simulink model "case7"  (R2024b)
settings: Solver=FixedStepAuto  StartTime=0  StopTime=1  FixedStep=1e-7  RelTol=1e-3
values from neighbouring files (symbols this model uses):
  SG_D_1_D = 0.01056    [IEEE9_case_parameters.m]    (also in case1_parameters.m; case2_parameters.m; case3_parameters.m; case4_parameters.m)
  SG_D_1_EnableSaturation = 0    [IEEE9_case_parameters.m]    (also in case1_parameters.m; case2_parameters.m; case3_parameters.m; case4_parameters.m)
  SG_D_1_f0 = 60    [IEEE9_case_parameters.m]    (also in case1_parameters.m; case2_parameters.m; case3_parameters.m; case4_parameters.m)
  SG_D_1_H = 7.5    [IEEE9_case_parameters.m]    (also in case1_parameters.m; case2_parameters.m; case3_parameters.m; case4_parameters.m)
  SG_D_1_K_A = 20    [IEEE9_case_parameters.m]    (also in case1_parameters.m; case2_parameters.m; case3_parameters.m; case4_parameters.m)
  SG_D_1_K_E = 1.000000e+1    (= 10)    [IEEE9_case_parameters.m]    (also in case1_parameters.m; case2_parameters.m; case3_parameters.m; case4_parameters.m)
  SG_D_1_K_F = 2.363    [IEEE9_case_parameters.m]    (also in case1_parameters.m; case2_parameters.m; case3_parameters.m; case4_parameters.m)
  SG_D_1_K_s = 0.5    [IEEE9_case_parameters.m]    (also in case1_parameters.m = 5; case2_parameters.m = 5; case3_parameters.m = 5; case4_parameters.m = 5)
  SG_D_1_R_a = 0.001088    [IEEE9_case_parameters.m]    (also in case1_parameters.m; case2_parameters.m; case3_parameters.m; case4_parameters.m)
  SG_D_1_S_A = 1    [IEEE9_case_parameters.m]    (also in case1_parameters.m; case2_parameters.m; case3_parameters.m; case4_parameters.m)
  SG_D_1_S_B = 0.103    [IEEE9_case_parameters.m]    (also in case1_parameters.m; case2_parameters.m; case3_parameters.m; case4_parameters.m)
  SG_D_1_S_N = 10.659857    [IEEE9_case_parameters.m]    (also in case1_parameters.m; case2_parameters.m; case3_parameters.m; case4_parameters.m)
  SG_D_1_SpeedPara = 200    [IEEE9_case_parameters.m]    (also in case1_parameters.m; case2_parameters.m; case3_parameters.m; case4_parameters.m)
  SG_D_1_T_0 = 0.720173    [IEEE9_case_parameters.m]    (also in case1_parameters.m = 0.755522; case2_parameters.m = 0.808931; case3_parameters.m = 0.869402; case4_parameters.m = 0.729316)
  SG_D_1_T_1 = 0.3    [IEEE9_case_parameters.m]    (also in case1_parameters.m; case2_parameters.m; case3_parameters.m; case4_parameters.m)
  SG_D_1_T_2 = 0.05    [IEEE9_case_parameters.m]    (also in case1_parameters.m; case2_parameters.m; case3_parameters.m; case4_parameters.m)
  SG_D_1_T_3 = 0.02    [IEEE9_case_parameters.m]    (also in case1_parameters.m; case2_parameters.m; case3_parameters.m; case4_parameters.m)
  SG_D_1_T_4 = 0.005    [IEEE9_case_parameters.m]    (also in case1_parameters.m; case2_parameters.m; case3_parameters.m; case4_parameters.m)
  SG_D_1_T_A = 0.02    [IEEE9_case_parameters.m]    (also in case1_parameters.m; case2_parameters.m; case3_parameters.m; case4_parameters.m)
  SG_D_1_T_dd = 8.000000e+0    (= 8)    [IEEE9_case_parameters.m]    (also in case1_parameters.m; case2_parameters.m; case3_parameters.m; case4_parameters.m)
  SG_D_1_T_ddd = 0.04    [IEEE9_case_parameters.m]    (also in case1_parameters.m; case2_parameters.m; case3_parameters.m; case4_parameters.m)
  SG_D_1_T_E = 0.314    [IEEE9_case_parameters.m]    (also in case1_parameters.m; case2_parameters.m; case3_parameters.m; case4_parameters.m)
  SG_D_1_T_F = 0.35    [IEEE9_case_parameters.m]    (also in case1_parameters.m; case2_parameters.m; case3_parameters.m; case4_parameters.m)
  SG_D_1_T_qd = 0.8    [IEEE9_case_parameters.m]    (also in case1_parameters.m; case2_parameters.m; case3_parameters.m; case4_parameters.m)
  SG_D_1_T_qdd = 0.02    [IEEE9_case_parameters.m]    (also in case1_parameters.m; case2_parameters.m; case3_parameters.m; case4_parameters.m)
  SG_D_1_T_speed = 0.1    [IEEE9_case_parameters.m]    (also in case1_parameters.m = 200; case2_parameters.m = 200; case3_parameters.m = 200; case4_parameters.m = 200)
  SG_D_1_T_w = 0.5    [IEEE9_case_parameters.m]    (also in case1_parameters.m; case2_parameters.m; case3_parameters.m; case4_parameters.m)
  SG_D_1_V_ref = 1.990276    [IEEE9_case_parameters.m]    (also in case1_parameters.m = 2.042296; case2_parameters.m = 2.051388; case3_parameters.m = 2.089584; case4_parameters.m = 2.01845)
  SG_D_1_w_ref = 376.991118    [IEEE9_case_parameters.m]    (also in case1_parameters.m; case2_parameters.m; case3_parameters.m; case4_parameters.m)
  SG_D_1_wb = 6.000000e+1    (= 60)    [IEEE9_case_parameters.m]    (also in case1_parameters.m; case2_parameters.m; case3_parameters.m; case4_parameters.m)
  SG_D_1_x_d = 1.9    [IEEE9_case_parameters.m]    (also in case1_parameters.m; case2_parameters.m; case3_parameters.m; case4_parameters.m)
  SG_D_1_x_dd = 0.302    [IEEE9_case_parameters.m]    (also in case1_parameters.m; case2_parameters.m; case3_parameters.m; case4_parameters.m)
  SG_D_1_x_ddd = 0.204    [IEEE9_case_parameters.m]    (also in case1_parameters.m; case2_parameters.m; case3_parameters.m; case4_parameters.m)
  SG_D_1_x_l = 0.05    [IEEE9_case_parameters.m]    (also in case1_parameters.m; case2_parameters.m; case3_parameters.m; case4_parameters.m)
  SG_D_1_x_q = 1.3    [IEEE9_case_parameters.m]    (also in case1_parameters.m; case2_parameters.m; case3_parameters.m; case4_parameters.m)
  SG_D_1_x_qd = 0.5    [IEEE9_case_parameters.m]    (also in case1_parameters.m; case2_parameters.m; case3_parameters.m; case4_parameters.m)
  SG_D_1_x_qdd = 0.3    [IEEE9_case_parameters.m]    (also in case1_parameters.m; case2_parameters.m; case3_parameters.m; case4_parameters.m)
  SG_D_2_D = 0.02    [IEEE9_case_parameters.m]    (also in case1_parameters.m; case2_parameters.m; case3_parameters.m; case4_parameters.m)
  SG_D_2_EnableSaturation = 0    [IEEE9_case_parameters.m]    (also in case1_parameters.m; case2_parameters.m; case3_parameters.m; case4_parameters.m)
  SG_D_2_f0 = 60    [IEEE9_case_parameters.m]    (also in case1_parameters.m; case2_parameters.m; case3_parameters.m; case4_parameters.m)
  SG_D_2_H = 8.000000e+0    (= 8)    [IEEE9_case_parameters.m]    (also in case1_parameters.m; case2_parameters.m; case3_parameters.m; case4_parameters.m)
  SG_D_2_K_A = 20    [IEEE9_case_parameters.m]    (also in case1_parameters.m; case2_parameters.m; case3_parameters.m; case4_parameters.m)
  SG_D_2_K_E = 1.000000e+1    (= 10)    [IEEE9_case_parameters.m]    (also in case1_parameters.m; case2_parameters.m; case3_parameters.m; case4_parameters.m)
  SG_D_2_K_F = 2.363    [IEEE9_case_parameters.m]    (also in case1_parameters.m; case2_parameters.m; case3_parameters.m; case4_parameters.m)
  SG_D_2_K_s = 0.5    [IEEE9_case_parameters.m]    (also in case1_parameters.m = 4; case2_parameters.m = 4; case3_parameters.m = 4; case4_parameters.m = 4)
  SG_D_2_R_a = 0.001088    [IEEE9_case_parameters.m]    (also in case1_parameters.m; case2_parameters.m; case3_parameters.m; case4_parameters.m)
  SG_D_2_S_A = 1    [IEEE9_case_parameters.m]    (also in case1_parameters.m; case2_parameters.m; case3_parameters.m; case4_parameters.m)
  SG_D_2_S_B = 0.103    [IEEE9_case_parameters.m]    (also in case1_parameters.m; case2_parameters.m; case3_parameters.m; case4_parameters.m)
  SG_D_2_S_N = 10.659857    [IEEE9_case_parameters.m]    (also in case1_parameters.m; case2_parameters.m; case3_parameters.m; case4_parameters.m)
  SG_D_2_SpeedPara = 200    [IEEE9_case_parameters.m]    (also in case1_parameters.m; case2_parameters.m; case3_parameters.m; case4_parameters.m)
  SG_D_2_T_0 = 1.632913    [IEEE9_case_parameters.m]    (also in case1_parameters.m = 1.632925; case2_parameters.m = 1.632915; case3_parameters.m = 1.632914; case4_parameters.m = 1.632927)
  SG_D_2_T_1 = 0.2    [IEEE9_case_parameters.m]    (also in case1_parameters.m; case2_parameters.m; case3_parameters.m; case4_parameters.m)
  SG_D_2_T_2 = 0.05    [IEEE9_case_parameters.m]    (also in case1_parameters.m; case2_parameters.m; case3_parameters.m; case4_parameters.m)
  SG_D_2_T_3 = 0.02    [IEEE9_case_parameters.m]    (also in case1_parameters.m; case2_parameters.m; case3_parameters.m; case4_parameters.m)
  SG_D_2_T_4 = 0.005    [IEEE9_case_parameters.m]    (also in case1_parameters.m; case2_parameters.m; case3_parameters.m; case4_parameters.m)
  SG_D_2_T_A = 0.02    [IEEE9_case_parameters.m]    (also in case1_parameters.m; case2_parameters.m; case3_parameters.m; case4_parameters.m)
  SG_D_2_T_dd = 7.9    [IEEE9_case_parameters.m]    (also in case1_parameters.m; case2_parameters.m; case3_parameters.m; case4_parameters.m)
  SG_D_2_T_ddd = 0.04    [IEEE9_case_parameters.m]    (also in case1_parameters.m; case2_parameters.m; case3_parameters.m; case4_parameters.m)
  SG_D_2_T_E = 0.314    [IEEE9_case_parameters.m]    (also in case1_parameters.m; case2_parameters.m; case3_parameters.m; case4_parameters.m)
  SG_D_2_T_F = 0.35    [IEEE9_case_parameters.m]    (also in case1_parameters.m; case2_parameters.m; case3_parameters.m; case4_parameters.m)
  SG_D_2_T_qd = 0.8    [IEEE9_case_parameters.m]    (also in case1_parameters.m; case2_parameters.m; case3_parameters.m; case4_parameters.m)
  SG_D_2_T_qdd = 0.015    [IEEE9_case_parameters.m]    (also in case1_parameters.m; case2_parameters.m; case3_parameters.m; case4_parameters.m)
  SG_D_2_T_speed = 0.1    [IEEE9_case_parameters.m]    (also in case1_parameters.m = 150; case2_parameters.m = 150; case3_parameters.m = 150; case4_parameters.m = 150)
  SG_D_2_T_w = 0.35    [IEEE9_case_parameters.m]    (also in case1_parameters.m; case2_parameters.m; case3_parameters.m; case4_parameters.m)
  SG_D_2_V_ref = 2.58547    [IEEE9_case_parameters.m]    (also in case1_parameters.m = 2.597896; case2_parameters.m = 2.587136; case3_parameters.m = 2.586042; case4_parameters.m = 2.599679)
  SG_D_2_w_ref = 376.991118    [IEEE9_case_parameters.m]    (also in case1_parameters.m; case2_parameters.m; case3_parameters.m; case4_parameters.m)
  SG_D_2_wb = 6.000000e+1    (= 60)    [IEEE9_case_parameters.m]    (also in case1_parameters.m; case2_parameters.m; case3_parameters.m; case4_parameters.m)
  SG_D_2_x_d = 1.8    [IEEE9_case_parameters.m]    (also in case1_parameters.m; case2_parameters.m; case3_parameters.m; case4_parameters.m)
  SG_D_2_x_dd = 0.302    [IEEE9_case_parameters.m]    (also in case1_parameters.m; case2_parameters.m; case3_parameters.m; case4_parameters.m)
  SG_D_2_x_ddd = 0.204    [IEEE9_case_parameters.m]    (also in case1_parameters.m; case2_parameters.m; case3_parameters.m; case4_parameters.m)
  SG_D_2_x_l = 0.05    [IEEE9_case_parameters.m]    (also in case1_parameters.m; case2_parameters.m; case3_parameters.m; case4_parameters.m)
  SG_D_2_x_q = 1.25    [IEEE9_case_parameters.m]    (also in case1_parameters.m; case2_parameters.m; case3_parameters.m; case4_parameters.m)
  SG_D_2_x_qd = 0.5    [IEEE9_case_parameters.m]    (also in case1_parameters.m; case2_parameters.m; case3_parameters.m; case4_parameters.m)
  SG_D_2_x_qdd = 0.3    [IEEE9_case_parameters.m]    (also in case1_parameters.m; case2_parameters.m; case3_parameters.m; case4_parameters.m)
  SG_D_3_D = 0.02    [IEEE9_case_parameters.m]    (also in case1_parameters.m; case2_parameters.m; case3_parameters.m; case4_parameters.m)
  SG_D_3_EnableSaturation = 0    [IEEE9_case_parameters.m]    (also in case1_parameters.m; case2_parameters.m; case3_parameters.m; case4_parameters.m)
  SG_D_3_f0 = 60    [IEEE9_case_parameters.m]    (also in case1_parameters.m; case2_parameters.m; case3_parameters.m; case4_parameters.m)
  SG_D_3_H = 7.7    [IEEE9_case_parameters.m]    (also in case1_parameters.m; case2_parameters.m; case3_parameters.m; case4_parameters.m)
  SG_D_3_K_A = 20    [IEEE9_case_parameters.m]    (also in case1_parameters.m; case2_parameters.m; case3_parameters.m; case4_parameters.m)
  SG_D_3_K_E = 1.000000e+1    (= 10)    [IEEE9_case_parameters.m]    (also in case1_parameters.m; case2_parameters.m; case3_parameters.m; case4_parameters.m)
  SG_D_3_K_F = 2.363    [IEEE9_case_parameters.m]    (also in case1_parameters.m; case2_parameters.m; case3_parameters.m; case4_parameters.m)
  SG_D_3_K_s = 0.2    [IEEE9_case_parameters.m]    (also in case1_parameters.m = 2; case2_parameters.m = 2; case3_parameters.m = 2; case4_parameters.m = 2)
  SG_D_3_R_a = 0.001088    [IEEE9_case_parameters.m]    (also in case1_parameters.m; case2_parameters.m; case3_parameters.m; case4_parameters.m)
  SG_D_3_S_A = 1    [IEEE9_case_parameters.m]    (also in case1_parameters.m; case2_parameters.m; case3_parameters.m; case4_parameters.m)
  SG_D_3_S_B = 0.103    [IEEE9_case_parameters.m]    (also in case1_parameters.m; case2_parameters.m; case3_parameters.m; case4_parameters.m)
  SG_D_3_S_N = 10.659857    [IEEE9_case_parameters.m]    (also in case1_parameters.m; case2_parameters.m; case3_parameters.m; case4_parameters.m)
  SG_D_3_SpeedPara = 200    [IEEE9_case_parameters.m]    (also in case1_parameters.m; case2_parameters.m; case3_parameters.m; case4_parameters.m)
  SG_D_3_T_0 = 0.850788    [IEEE9_case_parameters.m]    (also in case1_parameters.m = 0.850786; case2_parameters.m = 0.850787; case3_parameters.m; case4_parameters.m = 0.850786)
  SG_D_3_T_1 = 0.2    [IEEE9_case_parameters.m]    (also in case1_parameters.m; case2_parameters.m; case3_parameters.m; case4_parameters.m)
  SG_D_3_T_2 = 0.05    [IEEE9_case_parameters.m]    (also in case1_parameters.m; case2_parameters.m; case3_parameters.m; case4_parameters.m)
  SG_D_3_T_3 = 0.02    [IEEE9_case_parameters.m]    (also in case1_parameters.m; case2_parameters.m; case3_parameters.m; case4_parameters.m)
  SG_D_3_T_4 = 0.005    [IEEE9_case_parameters.m]    (also in case1_parameters.m; case2_parameters.m; case3_parameters.m; case4_parameters.m)
  SG_D_3_T_A = 0.02    [IEEE9_case_parameters.m]    (also in case1_parameters.m; case2_parameters.m; case3_parameters.m; case4_parameters.m)
  SG_D_3_T_dd = 8.1    [IEEE9_case_parameters.m]    (also in case1_parameters.m; case2_parameters.m; case3_parameters.m; case4_parameters.m)
  SG_D_3_T_ddd = 0.04    [IEEE9_case_parameters.m]    (also in case1_parameters.m; case2_parameters.m; case3_parameters.m; case4_parameters.m)
  SG_D_3_T_E = 0.314    [IEEE9_case_parameters.m]    (also in case1_parameters.m; case2_parameters.m; case3_parameters.m; case4_parameters.m)
  SG_D_3_T_F = 0.35    [IEEE9_case_parameters.m]    (also in case1_parameters.m; case2_parameters.m; case3_parameters.m; case4_parameters.m)
  SG_D_3_T_qd = 0.8    [IEEE9_case_parameters.m]    (also in case1_parameters.m; case2_parameters.m; case3_parameters.m; case4_parameters.m)
  SG_D_3_T_qdd = 0.015    [IEEE9_case_parameters.m]    (also in case1_parameters.m; case2_parameters.m; case3_parameters.m; case4_parameters.m)
  SG_D_3_T_speed = 0.1    [IEEE9_case_parameters.m]    (also in case1_parameters.m = 180; case2_parameters.m = 180; case3_parameters.m = 180; case4_parameters.m = 180)
  SG_D_3_T_w = 0.4    [IEEE9_case_parameters.m]    (also in case1_parameters.m; case2_parameters.m; case3_parameters.m; case4_parameters.m)
  SG_D_3_V_ref = 1.892727    [IEEE9_case_parameters.m]    (also in case1_parameters.m = 1.906439; case2_parameters.m = 1.895535; case3_parameters.m = 1.892105; case4_parameters.m = 1.906598)
  SG_D_3_w_ref = 376.991118    [IEEE9_case_parameters.m]    (also in case1_parameters.m; case2_parameters.m; case3_parameters.m; case4_parameters.m)
  SG_D_3_wb = 6.000000e+1    (= 60)    [IEEE9_case_parameters.m]    (also in case1_parameters.m; case2_parameters.m; case3_parameters.m; case4_parameters.m)
  SG_D_3_x_d = 1.85    [IEEE9_case_parameters.m]    (also in case1_parameters.m; case2_parameters.m; case3_parameters.m; case4_parameters.m)
  SG_D_3_x_dd = 0.302    [IEEE9_case_parameters.m]    (also in case1_parameters.m; case2_parameters.m; case3_parameters.m; case4_parameters.m)
  SG_D_3_x_ddd = 0.204    [IEEE9_case_parameters.m]    (also in case1_parameters.m; case2_parameters.m; case3_parameters.m; case4_parameters.m)
  SG_D_3_x_l = 0.05    [IEEE9_case_parameters.m]    (also in case1_parameters.m; case2_parameters.m; case3_parameters.m; case4_parameters.m)
  SG_D_3_x_q = 1.2    [IEEE9_case_parameters.m]    (also in case1_parameters.m; case2_parameters.m; case3_parameters.m; case4_parameters.m)
  SG_D_3_x_qd = 0.5    [IEEE9_case_parameters.m]    (also in case1_parameters.m; case2_parameters.m; case3_parameters.m; case4_parameters.m)
  SG_D_3_x_qdd = 0.3    [IEEE9_case_parameters.m]    (also in case1_parameters.m; case2_parameters.m; case3_parameters.m; case4_parameters.m)
(part 7 of 12)

== system case7/SG_D_2/T_e_SG_D_2_block ==
  note: T_e_SG_D_2 in case7
      | $-\frac{\psi _{d,\mathrm{SG},D,2}\,\left(\psi _{q,\mathrm{SG},D,2}+\frac{\psi _{\mathrm{gq},\mathrm{SG},D,2}\,\left(x_{l}-x_{\mathrm{qdd}}\right)}{x_{l}-x_{\mathrm{qd}}}+\frac{\psi _{\mathrm{kq},\mathrm{SG},D,2}\,\left(x_{\mathrm{qd}}-x_{\mathrm{qdd}}\right)}{x_{l}-x_{\mathrm{qd}}}\right)}{x_{\mathrm{qdd}}}-\frac{\psi _{q,\mathrm{SG},D,2}\,\left(\frac{\psi _{\mathrm{1d},\mathrm{SG},D,2}\,\left(x_{\mathrm{dd}}-x_{\mathrm{ddd}}\right)}{x_{\mathrm{dd}}-x_{l}}-\psi _{d,\mathrm{SG},D,2}+\frac{\psi _{\mathrm{fd},\mathrm{SG},D,2}\,\left(x_{\mathrm{ddd}}-x_{l}\right)}{x_{\mathrm{dd}}-x_{l}}\right)}{x_{\mathrm{ddd}}}$
      | Automatically generated on 2025-10-31 19:25:20 .
  State_psi_d_SG_D_2_bf269 : Inport
  State_psi_gq_SG_D_2_7da5e : Inport  Port=2
  State_psi_kq_SG_D_2_7391f : Inport  Port=3
  State_psi_q_SG_D_2_f6431 : Inport  Port=4
  State_psi_q_SG_D_2_7a09c : Inport  Port=5
  State_psi_1d_SG_D_2_55ddd : Inport  Port=6
  State_psi_d_SG_D_2_ae3de : Inport  Port=7
  State_psi_fd_SG_D_2_f8f9e : Inport  Port=8
  Add_2b13d : Sum
  Add_36812 : Sum
  Add_50ba8 : Sum
  Add_580a7 : Sum
  Add_7cac4 : Sum
  Add_a9295 : Sum
  Constant_-1_2379d : Constant  Value=-1
  Constant_-1_707ee : Constant  Value=-1
  Constant_-1_ac65e : Constant  Value=-1
  Constant_-1_e5db3 : Constant  Value=-1
  Constant_-1_f398b : Constant  Value=-1
  Constant_x_dd_0d9b9 : Constant  Value=x_dd
  Constant_x_dd_25ccc : Constant  Value=x_dd
  Constant_x_dd_6eda6 : Constant  Value=x_dd
  Constant_x_ddd_00b35 : Constant  Value=x_ddd
  Constant_x_ddd_04d20 : Constant  Value=x_ddd
  Constant_x_ddd_4eb00 : Constant  Value=x_ddd
  Constant_x_l_21d65 : Constant  Value=x_l
  Constant_x_l_63637 : Constant  Value=x_l
  Constant_x_l_ad282 : Constant  Value=x_l
  Constant_x_l_d3278 : Constant  Value=x_l
  Constant_x_l_e1734 : Constant  Value=x_l
  Constant_x_l_f33b5 : Constant  Value=x_l
  Constant_x_qd_230c4 : Constant  Value=x_qd
  Constant_x_qd_85d67 : Constant  Value=x_qd
  Constant_x_qd_c57f3 : Constant  Value=x_qd
  Constant_x_qdd_b2a71 : Constant  Value=x_qdd
  Constant_x_qdd_e14ff : Constant  Value=x_qdd
  Constant_x_qdd_e3c02 : Constant  Value=x_qdd
  Divide_2619b : Product  Inputs=*/
  Divide_6dcfa : Product  Inputs=*/
  Divide_a7b51 : Product  Inputs=*/
  Divide_e1466 : Product  Inputs=*/
  Divide_fc8fb : Product  Inputs=*/
  Divide_fe27d : Product  Inputs=*/
  Product_015a5 : Product
  Product_21805 : Product
  Product_3d83f : Product
  Product_420f9 : Product
  Product_4241e : Product
  Product_5588b : Product
  Product_61e6b : Product
  Product_98e5c : Product
  Product_d02a4 : Product
  Product_e1847 : Product
  Product_e3d6a : Product
  Subtract_2dfcc : Sum  Inputs=+-
  Subtract_2ef2d : Sum  Inputs=+-
  Subtract_4663c : Sum  Inputs=+-
  Subtract_4e099 : Sum  Inputs=+-
  Subtract_9b5ee : Sum  Inputs=+-
  Subtract_f4c7b : Sum  Inputs=+-
  Subtract_f8d72 : Sum  Inputs=+-
  Blockout_T_e_SG_D_2_730cc : Outport
  wires:
  Constant_-1_f398b/1 -> Product_21805/1
  Divide_a7b51/1 -> Subtract_f8d72/1
  Constant_-1_707ee/1 -> Product_3d83f/1
  Constant_x_l_21d65/1 -> Product_3d83f/2
  Constant_x_qd_c57f3/1 -> Subtract_2ef2d/1
  Product_61e6b/1 -> Divide_a7b51/1
  Product_3d83f/1 -> Add_a9295/1
  Divide_6dcfa/1 -> Subtract_4e099/2
  Constant_x_qdd_e14ff/1 -> Subtract_2ef2d/2
  Constant_x_qdd_b2a71/1 -> Divide_e1466/2
  Constant_x_ddd_04d20/1 -> Subtract_9b5ee/2
  Constant_x_qdd_e3c02/1 -> Add_a9295/2
  Constant_x_l_e1734/1 -> Product_21805/2
  Constant_-1_e5db3/1 -> Product_98e5c/1
  Constant_x_l_63637/1 -> Product_98e5c/2
  Constant_-1_ac65e/1 -> Product_5588b/1
  State_psi_1d_SG_D_2_55ddd/1 -> Product_5588b/2
  Constant_x_dd_25ccc/1 -> Subtract_9b5ee/1
  Divide_fe27d/1 -> Subtract_f8d72/2
  State_psi_gq_SG_D_2_7da5e/1 -> Product_61e6b/1
  Add_a9295/1 -> Product_61e6b/2
  Subtract_f8d72/1 -> Add_580a7/1
  Constant_x_dd_6eda6/1 -> Subtract_f4c7b/1
  Product_21805/1 -> Add_7cac4/1
  Product_015a5/1 -> Product_e1847/1
  Constant_x_qd_85d67/1 -> Add_7cac4/2
  State_psi_kq_SG_D_2_7391f/1 -> Product_420f9/1
  Subtract_2ef2d/1 -> Product_420f9/2
  Product_98e5c/1 -> Add_2b13d/1
  State_psi_q_SG_D_2_7a09c/1 -> Product_d02a4/1
  Constant_x_qd_230c4/1 -> Add_2b13d/2
  Product_5588b/1 -> Product_e3d6a/1
  Divide_fc8fb/1 -> Add_50ba8/2
  Subtract_9b5ee/1 -> Product_e3d6a/2
  Constant_x_l_f33b5/1 -> Subtract_f4c7b/2
  Constant_x_ddd_4eb00/1 -> Subtract_2dfcc/1
  Constant_x_dd_0d9b9/1 -> Subtract_4663c/1
  Constant_x_l_ad282/1 -> Subtract_2dfcc/2
  Add_50ba8/1 -> Blockout_T_e_SG_D_2_730cc/1
  Add_7cac4/1 -> Divide_a7b51/2
  Product_420f9/1 -> Divide_fe27d/1
  Product_e1847/1 -> Divide_e1466/1
  State_psi_d_SG_D_2_bf269/1 -> Product_015a5/2
  Add_2b13d/1 -> Divide_fe27d/2
  Product_e3d6a/1 -> Divide_2619b/1
  Subtract_f4c7b/1 -> Divide_2619b/2
  Constant_x_l_d3278/1 -> Subtract_4663c/2
  State_psi_fd_SG_D_2_f8f9e/1 -> Product_4241e/1
  Constant_x_ddd_00b35/1 -> Divide_fc8fb/2
  Product_d02a4/1 -> Divide_fc8fb/1
  Subtract_2dfcc/1 -> Product_4241e/2
  Divide_2619b/1 -> Add_36812/1
  State_psi_d_SG_D_2_ae3de/1 -> Add_36812/2
  Add_36812/1 -> Subtract_4e099/1
  Product_4241e/1 -> Divide_6dcfa/1
  Subtract_4663c/1 -> Divide_6dcfa/2
  Constant_-1_2379d/1 -> Product_015a5/1
  State_psi_q_SG_D_2_f6431/1 -> Add_580a7/2
  Add_580a7/1 -> Product_e1847/2
  Subtract_4e099/1 -> Product_d02a4/2
  Divide_e1466/1 -> Add_50ba8/1

== system case7/SG_D_2/d_E_fd_SG_D_2_block ==
  note: d_E_fd_SG_D_2 in case7
      | $\frac{V_{f,\mathrm{SG},D,2}-E_{\mathrm{fd},\mathrm{SG},D,2}\,K_{E}}{T_{E}}$
      | Automatically generated on 2025-10-31 19:25:00 .
  State_E_fd_SG_D_2_ac2d4 : Inport
  State_V_f_SG_D_2_83e9f : Inport  Port=2
  Add_7bd4d : Sum
  Constant_-1_a534e : Constant  Value=-1
  Constant_K_E_63bf6 : Constant  Value=K_E
  Constant_T_E_208ee : Constant  Value=T_E
  Divide_0c54f : Product  Inputs=*/
  Product_1a30a : Product
  Product_582a9 : Product
  Blockout_d_E_fd_SG_D_2_7fc5f : Outport
  wires:
  Constant_-1_a534e/1 -> Product_1a30a/1
  State_E_fd_SG_D_2_ac2d4/1 -> Product_1a30a/2
  Product_1a30a/1 -> Product_582a9/1
  Constant_K_E_63bf6/1 -> Product_582a9/2
  Product_582a9/1 -> Add_7bd4d/1
  Constant_T_E_208ee/1 -> Divide_0c54f/2
  State_V_f_SG_D_2_83e9f/1 -> Add_7bd4d/2
  Add_7bd4d/1 -> Divide_0c54f/1
  Divide_0c54f/1 -> Blockout_d_E_fd_SG_D_2_7fc5f/1

== system case7/SG_D_2/d_Px_1_SG_D_2_block ==
  note: d_Px_1_SG_D_2 in case7
      | $\frac{w_{\mathrm{SG},D,2}-2\,\pi \,f_{0}}{T_{w}}-\frac{\mathrm{Px}_{1,\mathrm{SG},D,2}}{T_{w}}$
      | Automatically generated on 2025-10-31 19:25:01 .
  State_Px_1_SG_D_2_f4101 : Inport
  State_w_SG_D_2_7a34c : Inport  Port=2
  Add_85e03 : Sum
  Add_c036b : Sum
  Constant_-1_0aa0c : Constant  Value=-1
  Constant_-2.0_febb9 : Constant  Value=-2.0
  Constant_T_w_270a6 : Constant  Value=T_w
  Constant_T_w_698d7 : Constant  Value=T_w
  Constant_f0_b5d65 : Constant  Value=f0
  Constant_pi_31b70 : Constant  Value=pi
  Divide_03843 : Product  Inputs=*/
  Divide_d2841 : Product  Inputs=*/
  Product_4a629 : Product
  Product_8553b : Product
  Product_cc20a : Product
  Blockout_d_Px_1_SG_D_2_2c2a9 : Outport
  wires:
  Constant_-2.0_febb9/1 -> Product_cc20a/1
  State_w_SG_D_2_7a34c/1 -> Add_c036b/2
  Constant_pi_31b70/1 -> Product_cc20a/2
  Product_cc20a/1 -> Product_8553b/1
  Constant_f0_b5d65/1 -> Product_8553b/2
  Constant_-1_0aa0c/1 -> Product_4a629/1
  State_Px_1_SG_D_2_f4101/1 -> Product_4a629/2
  Product_8553b/1 -> Add_c036b/1
  Product_4a629/1 -> Divide_03843/1
  Constant_T_w_698d7/1 -> Divide_03843/2
  Add_c036b/1 -> Divide_d2841/1
  Constant_T_w_270a6/1 -> Divide_d2841/2
  Divide_03843/1 -> Add_85e03/1
  Divide_d2841/1 -> Add_85e03/2
  Add_85e03/1 -> Blockout_d_Px_1_SG_D_2_2c2a9/1

== system case7/SG_D_2/d_Px_2_SG_D_2_block ==
  note: d_Px_2_SG_D_2 in case7
      | $\frac{\mathrm{Px}_{1,\mathrm{SG},D,2}-T_{2}\,\left(\frac{\mathrm{Px}_{1,\mathrm{SG},D,2}}{T_{w}}-\frac{w_{\mathrm{SG},D,2}-2\,\pi \,f_{0}}{T_{w}}\right)}{T_{1}}-\frac{\mathrm{Px}_{2,\mathrm{SG},D,2}}{T_{1}}$
      | Automatically generated on 2025-10-31 19:25:03 .
  State_Px_2_SG_D_2_9a1df : Inport
  State_Px_1_SG_D_2_e97bf : Inport  Port=2
  State_Px_1_SG_D_2_8c4e1 : Inport  Port=3
  State_w_SG_D_2_465a1 : Inport  Port=4
  Add_5cba5 : Sum
  Add_a3324 : Sum
  Add_cd739 : Sum
  Add_f40a7 : Sum
  Constant_-1_6e2c8 : Constant  Value=-1
  Constant_-1_ca048 : Constant  Value=-1
  Constant_-2.0_caa65 : Constant  Value=-2.0
  Constant_T_1_4ba06 : Constant  Value=T_1
  Constant_T_1_77ef5 : Constant  Value=T_1
  Constant_T_2_4bb2f : Constant  Value=T_2
  Constant_T_w_97444 : Constant  Value=T_w
  Constant_T_w_bf9f9 : Constant  Value=T_w
  Constant_f0_b11e2 : Constant  Value=f0
  Constant_pi_17818 : Constant  Value=pi
  Divide_2f8f1 : Product  Inputs=*/
  Divide_9a72a : Product  Inputs=*/
  Divide_a7fe4 : Product  Inputs=*/
  Divide_c8e5d : Product  Inputs=*/
  Product_2e68b : Product
  Product_83589 : Product
  Product_b2f5f : Product
  Product_d7499 : Product
  Product_ee69f : Product
  Blockout_d_Px_2_SG_D_2_f4188 : Outport
  wires:
  Constant_-1_6e2c8/1 -> Product_83589/1
  Constant_-2.0_caa65/1 -> Product_d7499/1
  Product_2e68b/1 -> Add_cd739/2
  State_w_SG_D_2_465a1/1 -> Add_5cba5/2
  Constant_pi_17818/1 -> Product_d7499/2
  Product_d7499/1 -> Product_ee69f/1
  State_Px_1_SG_D_2_8c4e1/1 -> Product_b2f5f/2
  Constant_f0_b11e2/1 -> Product_ee69f/2
  State_Px_2_SG_D_2_9a1df/1 -> Product_83589/2
  Constant_-1_ca048/1 -> Product_b2f5f/1
  Product_ee69f/1 -> Add_5cba5/1
  Product_b2f5f/1 -> Divide_2f8f1/1
  Constant_T_w_97444/1 -> Divide_2f8f1/2
  Add_5cba5/1 -> Divide_c8e5d/1
  Constant_T_w_bf9f9/1 -> Divide_c8e5d/2
  Divide_2f8f1/1 -> Add_a3324/1
  Divide_c8e5d/1 -> Add_a3324/2
  Constant_T_2_4bb2f/1 -> Product_2e68b/1
  Add_a3324/1 -> Product_2e68b/2
  State_Px_1_SG_D_2_e97bf/1 -> Add_cd739/1
  Product_83589/1 -> Divide_a7fe4/1
  Constant_T_1_77ef5/1 -> Divide_a7fe4/2
  Add_cd739/1 -> Divide_9a72a/1
  Constant_T_1_4ba06/1 -> Divide_9a72a/2
  Divide_a7fe4/1 -> Add_f40a7/1
  Divide_9a72a/1 -> Add_f40a7/2
  Add_f40a7/1 -> Blockout_d_Px_2_SG_D_2_f4188/1

== system case7/SG_D_2/d_Px_3_SG_D_2_block ==
  note: d_Px_3_SG_D_2 in case7
      | $\frac{\mathrm{Px}_{2,\mathrm{SG},D,2}+T_{4}\,\left(\frac{\mathrm{Px}_{1,\mathrm{SG},D,2}-T_{2}\,\left(\frac{\mathrm{Px}_{1,\mathrm{SG},D,2}}{T_{w}}-\frac{w_{\mathrm{SG},D,2}-2\,\pi \,f_{0}}{T_{w}}\right)}{T_{1}}-\frac{\mathrm{Px}_{2,\mathrm{SG},D,2}}{T_{1}}\right)}{T_{3}}-\frac{\mathrm{Px}_{3,\mathrm{SG},D,2}}{T_{3}}$
      | Automatically generated on 2025-10-31 19:25:06 .
  State_Px_3_SG_D_2_9d0f6 : Inport
  State_Px_2_SG_D_2_71991 : Inport  Port=2
  State_Px_2_SG_D_2_f02e6 : Inport  Port=3
  State_Px_1_SG_D_2_7e74e : Inport  Port=4
  State_Px_1_SG_D_2_1642d : Inport  Port=5
  State_w_SG_D_2_022fa : Inport  Port=6
  Add_0a98f : Sum
  Add_3fa49 : Sum
  Add_673a9 : Sum
  Add_a22dd : Sum
  Add_ad8a0 : Sum
  Add_f6a2a : Sum
  Constant_-1_1c951 : Constant  Value=-1
  Constant_-1_23c9e : Constant  Value=-1
  Constant_-1_88d62 : Constant  Value=-1
  Constant_-2.0_75075 : Constant  Value=-2.0
  Constant_T_1_10692 : Constant  Value=T_1
  Constant_T_1_1c2ec : Constant  Value=T_1
  Constant_T_2_aea25 : Constant  Value=T_2
  Constant_T_3_0ec24 : Constant  Value=T_3
  Constant_T_3_10ee6 : Constant  Value=T_3
  Constant_T_4_ef85c : Constant  Value=T_4
  Constant_T_w_03458 : Constant  Value=T_w
  Constant_T_w_d6821 : Constant  Value=T_w
  Constant_f0_5ab2a : Constant  Value=f0
  Constant_pi_85b82 : Constant  Value=pi
  Divide_03b6f : Product  Inputs=*/
  Divide_18901 : Product  Inputs=*/
  Divide_2be40 : Product  Inputs=*/
  Divide_35c63 : Product  Inputs=*/
  Divide_bf56f : Product  Inputs=*/
  Divide_f5027 : Product  Inputs=*/
  Product_211f0 : Product
  Product_35b53 : Product
  Product_668ab : Product
  Product_8a2c3 : Product
  Product_9009f : Product
  Product_d9840 : Product
  Product_e21ce : Product
  Blockout_d_Px_3_SG_D_2_173a6 : Outport
  wires:
  Constant_-2.0_75075/1 -> Product_668ab/1
  State_w_SG_D_2_022fa/1 -> Add_3fa49/2
  Add_f6a2a/1 -> Divide_f5027/1
  Constant_pi_85b82/1 -> Product_668ab/2
  Constant_-1_88d62/1 -> Product_9009f/1
  Product_668ab/1 -> Product_35b53/1
  State_Px_2_SG_D_2_f02e6/1 -> Product_9009f/2
  State_Px_1_SG_D_2_1642d/1 -> Product_8a2c3/2
  Divide_f5027/1 -> Add_a22dd/2
  Constant_f0_5ab2a/1 -> Product_35b53/2
  Constant_-1_1c951/1 -> Product_8a2c3/1
  Product_35b53/1 -> Add_3fa49/1
  Product_8a2c3/1 -> Divide_35c63/1
  Constant_T_w_d6821/1 -> Divide_35c63/2
  Divide_2be40/1 -> Add_a22dd/1
  Add_3fa49/1 -> Divide_03b6f/1
  Product_211f0/1 -> Add_0a98f/2
  Constant_T_w_03458/1 -> Divide_03b6f/2
  Divide_35c63/1 -> Add_673a9/1
  State_Px_1_SG_D_2_7e74e/1 -> Add_0a98f/1
  Divide_03b6f/1 -> Add_673a9/2
  Constant_-1_23c9e/1 -> Product_d9840/1
  Constant_T_2_aea25/1 -> Product_211f0/1
  Add_673a9/1 -> Product_211f0/2
  Product_9009f/1 -> Divide_18901/1
  Constant_T_1_10692/1 -> Divide_18901/2
  Add_0a98f/1 -> Divide_bf56f/1
  Constant_T_1_1c2ec/1 -> Divide_bf56f/2
  Divide_18901/1 -> Add_ad8a0/1
  Divide_bf56f/1 -> Add_ad8a0/2
  Constant_T_4_ef85c/1 -> Product_e21ce/1
  Add_ad8a0/1 -> Product_e21ce/2
  State_Px_3_SG_D_2_9d0f6/1 -> Product_d9840/2
  State_Px_2_SG_D_2_71991/1 -> Add_f6a2a/1
  Product_e21ce/1 -> Add_f6a2a/2
  Product_d9840/1 -> Divide_2be40/1
  Constant_T_3_0ec24/1 -> Divide_2be40/2
  Constant_T_3_10ee6/1 -> Divide_f5027/2
  Add_a22dd/1 -> Blockout_d_Px_3_SG_D_2_173a6/1

== system case7/SG_D_2/d_R_f_SG_D_2_block ==
  note: d_R_f_SG_D_2 in case7
      | $-\frac{R_{f,\mathrm{SG},D,2}-\frac{E_{\mathrm{fd},\mathrm{SG},D,2}\,K_{F}}{T_{F}}}{T_{F}}$
      | Automatically generated on 2025-10-31 19:24:59 .
  State_E_fd_SG_D_2_7a8b0 : Inport
  State_R_f_SG_D_2_2054a : Inport  Port=2
  Constant_K_F_8141e : Constant  Value=K_F
  Constant_T_F_69324 : Constant  Value=T_F
  Constant_T_F_9b1f8 : Constant  Value=T_F
  Divide_0f5e6 : Product  Inputs=*/
  Divide_31ab1 : Product  Inputs=*/
  Product_ef4c4 : Product
  Subtract_89368 : Sum  Inputs=+-
  Blockout_d_R_f_SG_D_2_b27f4 : Outport
  wires:
  Constant_T_F_9b1f8/1 -> Divide_31ab1/2
  State_E_fd_SG_D_2_7a8b0/1 -> Product_ef4c4/1
  Constant_K_F_8141e/1 -> Product_ef4c4/2
  State_R_f_SG_D_2_2054a/1 -> Subtract_89368/2
  Product_ef4c4/1 -> Divide_31ab1/1
  Divide_31ab1/1 -> Subtract_89368/1
  Constant_T_F_69324/1 -> Divide_0f5e6/2
  Subtract_89368/1 -> Divide_0f5e6/1
  Divide_0f5e6/1 -> Blockout_d_R_f_SG_D_2_b27f4/1

== system case7/SG_D_2/d_T_m_SG_D_2_block ==
  note: d_T_m_SG_D_2 in case7
      | $-\frac{T_{m,\mathrm{SG},D,2}-T_{0}+\frac{\mathrm{SpeedPara}\,\left(w_{\mathrm{SG},D,2}-w_{\mathrm{ref}}\right)}{2\,f_{0}\,\pi }}{T_{\mathrm{speed}}}$
      | Automatically generated on 2025-10-31 19:24:48 .
  State_w_SG_D_2_7be82 : Inport
  State_T_m_SG_D_2_01c83 : Inport  Port=2
  Add_59a2c : Sum
  Add_fa598 : Sum
  Constant_-1_1d92f : Constant  Value=-1
  Constant_2.0_9cf0c : Constant  Value=2.0
  Constant_SpeedPara_fea54 : Constant  Value=SpeedPara
  Constant_T_0_9e7ae : Constant  Value=T_0
  Constant_T_speed_a07ac : Constant  Value=T_speed
  Constant_f0_43f90 : Constant  Value=f0
  Constant_pi_a5e89 : Constant  Value=pi
  Constant_w_ref_b5b5c : Constant  Value=w_ref
  Divide_92970 : Product  Inputs=*/
  Divide_a6e8c : Product  Inputs=*/
  Product_02959 : Product
  Product_6d3a2 : Product
  Product_77f1d : Product
  Product_b372f : Product
  Subtract_b501a : Sum  Inputs=+-
  Blockout_d_T_m_SG_D_2_7fa4d : Outport
  wires:
  Constant_pi_a5e89/1 -> Product_6d3a2/2
  Constant_-1_1d92f/1 -> Product_77f1d/1
  Constant_w_ref_b5b5c/1 -> Add_fa598/2
  State_w_SG_D_2_7be82/1 -> Product_77f1d/2
  Product_77f1d/1 -> Add_fa598/1
  Add_59a2c/1 -> Subtract_b501a/1
  Add_fa598/1 -> Product_b372f/2
  Constant_2.0_9cf0c/1 -> Product_6d3a2/1
  Constant_SpeedPara_fea54/1 -> Product_b372f/1
  Product_6d3a2/1 -> Product_02959/1
  Constant_f0_43f90/1 -> Product_02959/2
  Product_b372f/1 -> Divide_92970/1
  Product_02959/1 -> Divide_92970/2
  Divide_92970/1 -> Add_59a2c/1
  Constant_T_0_9e7ae/1 -> Add_59a2c/2
  State_T_m_SG_D_2_01c83/1 -> Subtract_b501a/2
  Subtract_b501a/1 -> Divide_a6e8c/1
  Constant_T_speed_a07ac/1 -> Divide_a6e8c/2
  Divide_a6e8c/1 -> Blockout_d_T_m_SG_D_2_7fa4d/1

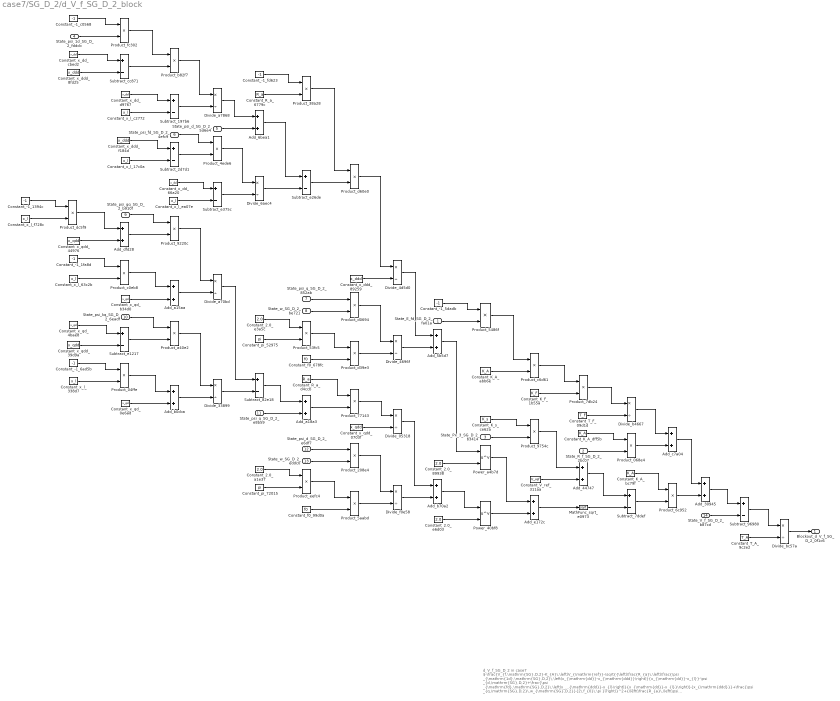
== system case7/SG_D_2/d_V_f_SG_D_2_block ==
  note: d_V_f_SG_D_2 in case7
      | $-\frac{V_{f,\mathrm{SG},D,2}-K_{A}\,\left(V_{\mathrm{ref}}-\sqrt{{\left(\frac{R_{a}\,\left(\frac{\psi _{\mathrm{1d},\mathrm{SG},D,2}\,\left(x_{\mathrm{dd}}-x_{\mathrm{ddd}}\right)}{x_{\mathrm{dd}}-x_{l}}-\psi _{d,\mathrm{SG},D,2}+\frac{\psi _{\mathrm{fd},\mathrm{SG},D,2}\,\left(x_{\mathrm{ddd}}-x_{l}\right)}{x_{\mathrm{dd}}-x_{l}}\right)}{x_{\mathrm{ddd}}}+\frac{\psi _{q,\mathrm{SG},D,2}\,w_{\mathrm{SG},D,2}}{2\,f_{0}\,\pi }\right)}^2+{\left(\frac{R_{a}\,\left(\psi _{q,\mathrm{SG},D,2}+\frac{\psi _{\mathrm{gq},\mathrm{SG},D,2}\,\left(x_{l}-x_{\mathrm{qdd}}\right)}{x_{l}-x_{\mathrm{qd}}}+\frac{\psi _{\mathrm{kq},\mathrm{SG},D,2}\,\left(x_{\mathrm{qd}}-x_{\mathrm{qdd}}\right)}{x_{l}-x_{\mathrm{qd}}}\right)}{x_{\mathrm{qdd}}}+\frac{\psi _{d,\mathrm{SG},D,2}\,w_{\mathrm{SG},D,2}}{2\,f_{0}\,\pi }\right)}^2}+K_{s}\,\mathrm{Px}_{3,\mathrm{SG},D,2}\right)-K_{A}\,R_{f,\mathrm{SG},D,2}+\frac{E_{\mathrm{fd},\mathrm{SG},D,2}\,K_{A}\,K_{F}}{T_{F}}}{T_{A}}$
      | Automatically generated on 2025-10-31 19:24:57 .
  State_E_fd_SG_D_2_fa01a : Inport
  State_R_f_SG_D_2_2bc07 : Inport  Port=2
  State_Px_3_SG_D_2_b3414 : Inport  Port=3
  State_psi_1d_SG_D_2_fddcb : Inport  Port=4
  State_psi_d_SG_D_2_5d6e4 : Inport  Port=5
  State_psi_fd_SG_D_2_4efc9 : Inport  Port=6
  State_psi_q_SG_D_2_852ab : Inport  Port=7
  State_w_SG_D_2_be721 : Inport  Port=8
  State_psi_gq_SG_D_2_b910f : Inport  Port=9
  State_psi_kq_SG_D_2_6eadf : Inport  Port=10
  State_psi_q_SG_D_2_e8b59 : Inport  Port=11
  State_psi_d_SG_D_2_e6df7 : Inport  Port=12
  State_w_SG_D_2_eddc0 : Inport  Port=13
  State_V_f_SG_D_2_b87cd : Inport  Port=14
  Add_30945 : Sum
  Add_44747 : Sum
  Add_5b5d7 : Sum
  Add_6bea1 : Sum
  Add_a15aa : Sum
  Add_a18a3 : Sum
  Add_b0cba : Sum
  Add_b70a2 : Sum
  Add_c7a04 : Sum
  Add_dfd28 : Sum
  Add_e172c : Sum
  Constant_-1_1394c : Constant  Value=-1
  Constant_-1_1fa8d : Constant  Value=-1
  Constant_-1_5dadb : Constant  Value=-1
  Constant_-1_6ad5b : Constant  Value=-1
  Constant_-1_c0568 : Constant  Value=-1
  Constant_-1_fd623 : Constant  Value=-1
  Constant_2.0_89938 : Constant  Value=2.0
  Constant_2.0_a1e37 : Constant  Value=2.0
  Constant_2.0_e3a5c : Constant  Value=2.0
  Constant_2.0_e6d03 : Constant  Value=2.0
  Constant_K_A_abb6e : Constant  Value=K_A
  Constant_K_A_bc79f : Constant  Value=K_A
  Constant_K_A_dff5b : Constant  Value=K_A
  Constant_K_F_1b55a : Constant  Value=K_F
  Constant_K_s_ce62a : Constant  Value=K_s
  Constant_R_a_6779c : Constant  Value=R_a
  Constant_R_a_d4ccb : Constant  Value=R_a
  Constant_T_A_9c2e2 : Constant  Value=T_A
  Constant_T_F_09d1d : Constant  Value=T_F
  Constant_V_ref_311aa : Constant  Value=V_ref
  Constant_f0_678fc : Constant  Value=f0
  Constant_f0_99d0a : Constant  Value=f0
  Constant_pi_52975 : Constant  Value=pi
  Constant_pi_72015 : Constant  Value=pi
  Constant_x_dd_66a20 : Constant  Value=x_dd
  Constant_x_dd_cbed2 : Constant  Value=x_dd
  Constant_x_dd_d9767 : Constant  Value=x_dd
  Constant_x_ddd_89259 : Constant  Value=x_ddd
  Constant_x_ddd_8fd25 : Constant  Value=x_ddd
  Constant_x_ddd_f184d : Constant  Value=x_ddd
  Constant_x_l_17c0a : Constant  Value=x_l
  Constant_x_l_338d7 : Constant  Value=x_l
  Constant_x_l_63c2b : Constant  Value=x_l
  Constant_x_l_c2772 : Constant  Value=x_l
  Constant_x_l_ea07e : Constant  Value=x_l
  Constant_x_l_f728c : Constant  Value=x_l
  Constant_x_qd_0e6ad : Constant  Value=x_qd
  Constant_x_qd_4bae8 : Constant  Value=x_qd
  Constant_x_qd_b34d0 : Constant  Value=x_qd
  Constant_x_qdd_0703f : Constant  Value=x_qdd
  Constant_x_qdd_39d9a : Constant  Value=x_qdd
  Constant_x_qdd_44976 : Constant  Value=x_qdd
  Divide_05318 : Product  Inputs=*/
  Divide_33899 : Product  Inputs=*/
  Divide_4696f : Product  Inputs=*/
  Divide_4d5d0 : Product  Inputs=*/
  Divide_6aec4 : Product  Inputs=*/
  Divide_a70bd : Product  Inputs=*/
  Divide_a7868 : Product  Inputs=*/
  Divide_b4667 : Product  Inputs=*/
  Divide_bc57a : Product  Inputs=*/
  Divide_f0e58 : Product  Inputs=*/
  MathFunc_sqrt_e0973 : Sqrt
  Power_40bf8 : Math  Operator=pow
  Power_a4b7d : Math  Operator=pow
  Product_04ffe : Product
  Product_068e4 : Product
  Product_208e4 : Product
  Product_38a28 : Product
  Product_4ede6 : Product
  Product_53fc5 : Product
  Product_5486f : Product
  Product_5aabd : Product
  Product_6c952 : Product
  Product_77143 : Product
  Product_7db24 : Product
  Product_9220c : Product
  Product_9754c : Product
  Product_a40e2 : Product
  Product_b82f7 : Product
  Product_c0eb8 : Product
  Product_c6d61 : Product
  Product_d0694 : Product
  Product_d39e3 : Product
  Product_d60e0 : Product
  Product_dc5f9 : Product
  Product_eefc4 : Product
  Product_fc302 : Product
  Subtract_197b6 : Sum  Inputs=+-
  Subtract_2d7d1 : Sum  Inputs=+-
  Subtract_7ddef : Sum  Inputs=+-
  Subtract_82e18 : Sum  Inputs=+-
  Subtract_96980 : Sum  Inputs=+-
  Subtract_cc871 : Sum  Inputs=+-
  Subtract_e1217 : Sum  Inputs=+-
  Subtract_e26de : Sum  Inputs=+-
  Subtract_e375c : Sum  Inputs=+-
  Blockout_d_V_f_SG_D_2_0f1c6 : Outport
  wires:
  Constant_-1_c0568/1 -> Product_fc302/1
  Constant_2.0_e3a5c/1 -> Product_53fc5/1
  Constant_-1_1394c/1 -> Product_dc5f9/1
  Product_53fc5/1 -> Product_d39e3/1
  Product_dc5f9/1 -> Add_dfd28/1
  Constant_x_l_338d7/1 -> Product_04ffe/2
  Constant_x_l_f728c/1 -> Product_dc5f9/2
  State_psi_1d_SG_D_2_fddcb/1 -> Product_fc302/2
  Constant_x_l_ea07e/1 -> Subtract_e375c/2
  Constant_x_dd_cbed2/1 -> Subtract_cc871/1
  Product_77143/1 -> Divide_05318/1
  Constant_x_ddd_8fd25/1 -> Subtract_cc871/2
  Constant_x_qd_0e6ad/1 -> Add_b0cba/2
  Add_dfd28/1 -> Product_9220c/2
  Constant_x_qdd_44976/1 -> Add_dfd28/2
  Constant_-1_1fa8d/1 -> Product_c0eb8/1
  Constant_x_dd_66a20/1 -> Subtract_e375c/1
  Subtract_82e18/1 -> Add_a18a3/1
  Power_a4b7d/1 -> Add_e172c/1
  Constant_x_l_63c2b/1 -> Product_c0eb8/2
  Constant_2.0_a1e37/1 -> Product_eefc4/1
  Constant_x_qd_4bae8/1 -> Subtract_e1217/1
  Constant_pi_72015/1 -> Product_eefc4/2
  Subtract_e26de/1 -> Product_d60e0/2
  Constant_x_qdd_39d9a/1 -> Subtract_e1217/2
  State_psi_fd_SG_D_2_4efc9/1 -> Product_4ede6/1
  Constant_-1_6ad5b/1 -> Product_04ffe/1
  Product_fc302/1 -> Product_b82f7/1
  State_w_SG_D_2_eddc0/1 -> Product_208e4/2
  Subtract_cc871/1 -> Product_b82f7/2
  Constant_x_dd_d9767/1 -> Subtract_197b6/1
  State_psi_q_SG_D_2_e8b59/1 -> Add_a18a3/2
  State_w_SG_D_2_be721/1 -> Product_d0694/2
  Subtract_2d7d1/1 -> Product_4ede6/2
  Constant_x_l_c2772/1 -> Subtract_197b6/2
  Add_c7a04/1 -> Add_30945/1
  Constant_x_ddd_f184d/1 -> Subtract_2d7d1/1
  Constant_x_l_17c0a/1 -> Subtract_2d7d1/2
  State_psi_gq_SG_D_2_b910f/1 -> Product_9220c/1
  Product_c0eb8/1 -> Add_a15aa/1
  Subtract_e375c/1 -> Divide_6aec4/2
  Constant_x_qd_b34d0/1 -> Add_a15aa/2
  Product_d0694/1 -> Divide_4696f/1
  State_psi_kq_SG_D_2_6eadf/1 -> Product_a40e2/1
  Subtract_e1217/1 -> Product_a40e2/2
  Product_4ede6/1 -> Divide_6aec4/1
  State_V_f_SG_D_2_b87cd/1 -> Subtract_96980/2
  Product_04ffe/1 -> Add_b0cba/1
  Product_b82f7/1 -> Divide_a7868/1
  Divide_a70bd/1 -> Subtract_82e18/1
  Subtract_197b6/1 -> Divide_a7868/2
  Product_9220c/1 -> Divide_a70bd/1
  Add_a15aa/1 -> Divide_a70bd/2
  Product_a40e2/1 -> Divide_33899/1
  Divide_6aec4/1 -> Subtract_e26de/2
  Constant_f0_678fc/1 -> Product_d39e3/2
  Add_b0cba/1 -> Divide_33899/2
  Divide_a7868/1 -> Add_6bea1/1
  State_psi_d_SG_D_2_5d6e4/1 -> Add_6bea1/2
  Divide_33899/1 -> Subtract_82e18/2
  Constant_-1_fd623/1 -> Product_38a28/1
  Constant_R_a_6779c/1 -> Product_38a28/2
  Constant_f0_99d0a/1 -> Product_5aabd/2
  Add_6bea1/1 -> Subtract_e26de/1
  Product_38a28/1 -> Product_d60e0/1
  Constant_pi_52975/1 -> Product_53fc5/2
  State_psi_q_SG_D_2_852ab/1 -> Product_d0694/1
  Constant_R_a_d4ccb/1 -> Product_77143/1
  State_E_fd_SG_D_2_fa01a/1 -> Product_5486f/2
  Add_a18a3/1 -> Product_77143/2
  State_psi_d_SG_D_2_e6df7/1 -> Product_208e4/1
  Product_eefc4/1 -> Product_5aabd/1
  Product_d60e0/1 -> Divide_4d5d0/1
  Constant_x_ddd_89259/1 -> Divide_4d5d0/2
  Product_d39e3/1 -> Divide_4696f/2
  Constant_x_qdd_0703f/1 -> Divide_05318/2
  Product_208e4/1 -> Divide_f0e58/1
  Product_5aabd/1 -> Divide_f0e58/2
  Divide_4d5d0/1 -> Add_5b5d7/1
  Divide_4696f/1 -> Add_5b5d7/2
  Divide_05318/1 -> Add_b70a2/1
  Divide_f0e58/1 -> Add_b70a2/2
  Constant_-1_5dadb/1 -> Product_5486f/1
  Add_5b5d7/1 -> Power_a4b7d/1
  Constant_2.0_89938/1 -> Power_a4b7d/2
  Add_b70a2/1 -> Power_40bf8/1
  Constant_2.0_e6d03/1 -> Power_40bf8/2
  Product_5486f/1 -> Product_c6d61/1
  Constant_K_A_abb6e/1 -> Product_c6d61/2
  Constant_K_s_ce62a/1 -> Product_9754c/1
  State_Px_3_SG_D_2_b3414/1 -> Product_9754c/2
  Power_40bf8/1 -> Add_e172c/2
  Product_c6d61/1 -> Product_7db24/1
  Constant_K_F_1b55a/1 -> Product_7db24/2
  Product_9754c/1 -> Add_44747/1
  Constant_V_ref_311aa/1 -> Add_44747/2
  Add_e172c/1 -> MathFunc_sqrt_e0973/1
  Product_7db24/1 -> Divide_b4667/1
  Constant_T_F_09d1d/1 -> Divide_b4667/2
  Constant_K_A_dff5b/1 -> Product_068e4/1
  State_R_f_SG_D_2_2bc07/1 -> Product_068e4/2
  Add_44747/1 -> Subtract_7ddef/1
  MathFunc_sqrt_e0973/1 -> Subtract_7ddef/2
  Divide_b4667/1 -> Add_c7a04/1
  Product_068e4/1 -> Add_c7a04/2
  Constant_K_A_bc79f/1 -> Product_6c952/1
  Subtract_7ddef/1 -> Product_6c952/2
  Product_6c952/1 -> Add_30945/2
  Add_30945/1 -> Subtract_96980/1
  Subtract_96980/1 -> Divide_bc57a/1
  Constant_T_A_9c2e2/1 -> Divide_bc57a/2
  Divide_bc57a/1 -> Blockout_d_V_f_SG_D_2_0f1c6/1

== system case7/SG_D_2/d_psi_1d_SG_D_2_block ==
  note: d_psi_1d_SG_D_2 in case7
      | $-\frac{\psi _{\mathrm{1d},\mathrm{SG},D,2}-\psi _{\mathrm{fd},\mathrm{SG},D,2}+\frac{\left(x_{\mathrm{dd}}-x_{l}\right)\,\left(\frac{\psi _{\mathrm{1d},\mathrm{SG},D,2}\,\left(x_{\mathrm{dd}}-x_{\mathrm{ddd}}\right)}{x_{\mathrm{dd}}-x_{l}}-\psi _{d,\mathrm{SG},D,2}+\frac{\psi _{\mathrm{fd},\mathrm{SG},D,2}\,\left(x_{\mathrm{ddd}}-x_{l}\right)}{x_{\mathrm{dd}}-x_{l}}\right)}{x_{\mathrm{ddd}}}}{T_{\mathrm{ddd}}}$
      | Automatically generated on 2025-10-31 19:24:27 .
  State_psi_1d_SG_D_2_3a9a3 : Inport
  State_psi_fd_SG_D_2_7f283 : Inport  Port=2
  State_psi_1d_SG_D_2_a8fff : Inport  Port=3
  State_psi_d_SG_D_2_2213a : Inport  Port=4
  State_psi_fd_SG_D_2_c6554 : Inport  Port=5
  Add_3b25f : Sum
  Add_baafb : Sum
  Add_ca49f : Sum
  Constant_-1_77da6 : Constant  Value=-1
  Constant_-1_b64dc : Constant  Value=-1
  Constant_T_ddd_aaf4e : Constant  Value=T_ddd
  Constant_x_dd_0aa91 : Constant  Value=x_dd
  Constant_x_dd_cc031 : Constant  Value=x_dd
  Constant_x_dd_d4f72 : Constant  Value=x_dd
  Constant_x_dd_dc41d : Constant  Value=x_dd
  Constant_x_ddd_141f6 : Constant  Value=x_ddd
  Constant_x_ddd_cd751 : Constant  Value=x_ddd
  Constant_x_ddd_e72f2 : Constant  Value=x_ddd
  Constant_x_l_2c965 : Constant  Value=x_l
  Constant_x_l_40d45 : Constant  Value=x_l
  Constant_x_l_998b9 : Constant  Value=x_l
  Constant_x_l_9fccf : Constant  Value=x_l
  Divide_08202 : Product  Inputs=*/
  Divide_9ca21 : Product  Inputs=*/
  Divide_e41b5 : Product  Inputs=*/
  Divide_ef371 : Product  Inputs=*/
  Product_3d170 : Product
  Product_47571 : Product
  Product_dc894 : Product
  Product_ef6c1 : Product
  Product_fc6e0 : Product
  Subtract_349ba : Sum  Inputs=+-
  Subtract_61169 : Sum  Inputs=+-
  Subtract_66282 : Sum  Inputs=+-
  Subtract_94a6a : Sum  Inputs=+-
  Subtract_9cd5e : Sum  Inputs=+-
  Subtract_a4d8a : Sum  Inputs=+-
  Blockout_d_psi_1d_SG_D_2_9a5fd : Outport
  wires:
  Subtract_61169/1 -> Product_fc6e0/2
  Constant_x_l_9fccf/1 -> Subtract_94a6a/2
  Divide_ef371/1 -> Add_ca49f/2
  Subtract_349ba/1 -> Product_dc894/2
  Constant_-1_b64dc/1 -> Product_3d170/1
  Constant_x_dd_d4f72/1 -> Subtract_a4d8a/1
  Divide_e41b5/1 -> Blockout_d_psi_1d_SG_D_2_9a5fd/1
  State_psi_fd_SG_D_2_7f283/1 -> Add_baafb/2
  State_psi_1d_SG_D_2_a8fff/1 -> Product_3d170/2
  Divide_9ca21/1 -> Subtract_349ba/2
  Constant_x_ddd_141f6/1 -> Subtract_a4d8a/2
  State_psi_1d_SG_D_2_3a9a3/1 -> Product_ef6c1/2
  Product_3d170/1 -> Product_47571/1
  Subtract_a4d8a/1 -> Product_47571/2
  Constant_x_dd_0aa91/1 -> Subtract_94a6a/1
  Constant_x_ddd_e72f2/1 -> Subtract_61169/1
  Constant_x_l_998b9/1 -> Subtract_61169/2
  Product_47571/1 -> Divide_08202/1
  Subtract_94a6a/1 -> Divide_08202/2
  State_psi_fd_SG_D_2_c6554/1 -> Product_fc6e0/1
  Constant_x_dd_dc41d/1 -> Subtract_9cd5e/1
  Constant_x_l_40d45/1 -> Subtract_66282/2
  Constant_x_l_2c965/1 -> Subtract_9cd5e/2
  Constant_x_ddd_cd751/1 -> Divide_ef371/2
  Divide_08202/1 -> Add_3b25f/1
  State_psi_d_SG_D_2_2213a/1 -> Add_3b25f/2
  Product_fc6e0/1 -> Divide_9ca21/1
  Subtract_9cd5e/1 -> Divide_9ca21/2
  Constant_x_dd_cc031/1 -> Subtract_66282/1
  Add_3b25f/1 -> Subtract_349ba/1
  Constant_-1_77da6/1 -> Product_ef6c1/1
  Subtract_66282/1 -> Product_dc894/1
  Product_ef6c1/1 -> Add_baafb/1
  Product_dc894/1 -> Divide_ef371/1
  Add_baafb/1 -> Add_ca49f/1
  Add_ca49f/1 -> Divide_e41b5/1
  Constant_T_ddd_aaf4e/1 -> Divide_e41b5/2
